simulink model "VendingMachine"  (R2018a)
settings: Solver=FixedStepDiscrete  StartTime=0.0  StopTime=1000  FixedStep=0.1  RelTol=1e-3  EnableMultiTasking=on
settings Model: Creator=higashit  LastModifiedBy=tliang
settings SolverCC: AlgebraicLoopSolver=LineSearch
settings DataIOCC: LimitDataPoints=on  SaveFormat=Array
settings OptimizationCC: DefaultParameterBehavior=Inlined  InlineInvariantSignals=on  ExpressionDepthLimit=2147483647  EfficientFloat2IntCast=on  LifeSpan=inf
settings DebuggingCC: SolverPrmCheckMsg=warning  UniqueDataStoreMsg=error  StateNameClashWarn=warning  StrictBusMsg=ErrorOnBusTreatedAsVector  SFUnexpectedBacktrackingDiag=warning  SFNoUnconditionalDefaultTransitionDiag=warning  SFExecutionAtInitializationDiag=none
settings HardwareCC: ProdBitPerPointer=32  ProdBitPerSizeT=32  ProdBitPerPtrDiffT=32  ProdLargestAtomicFloat=None  ProdIntDivRoundTo=Undefined  ProdEndianess=Unspecified  ProdWordSize=32  ProdHWDeviceType=32-bit Generic
settings ModelReferenceCC: PropagateSignalLabelsOutOfModel=off
settings CodeAppCC: StateflowObjectComments=on
settings GRTTargetCC: TargetLangStandard=C89/C90 (ANSI)  GeneratePreprocessorConditionals=Disable all
settings ConfigComp: CovMetricSettings=dw  CovHtmlReporting=on  CovSaveCumulativeToWorkspaceVar=on  CovSaveSingleToWorkspaceVar=on  CovExternalEMLEnable=off

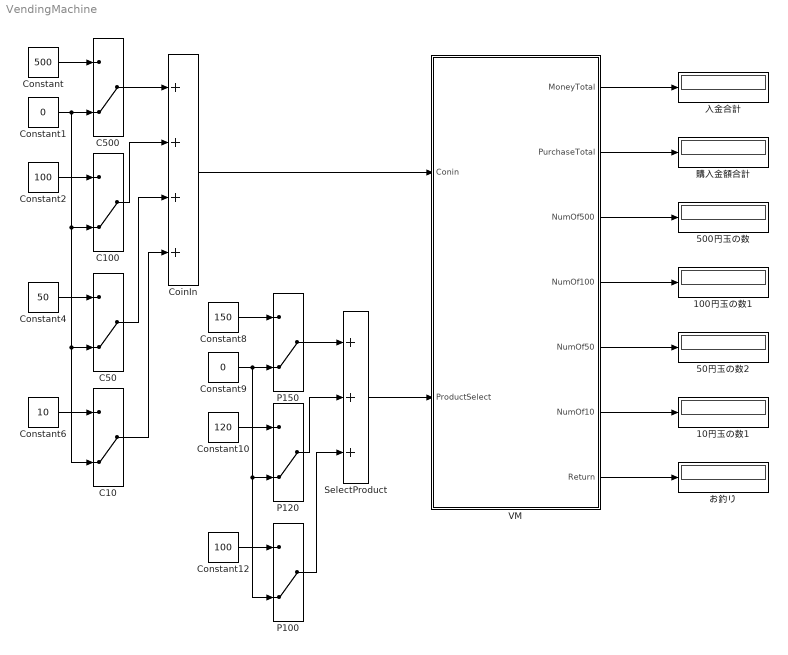
== system VendingMachine ==
  100円玉の数1 : Display
  10円玉の数1 : Display
  500円玉の数 : Display
  50円玉の数2 : Display
  C{10,50,100,500} (4 alike) : ManualSwitch  CurrentSetting=0
  CoinIn : Sum  Inputs=++++
  Constant : Constant  Value=500
  Constant1 : Constant  Value=0
  Constant10 : Constant  Value=120
  Constant12 : Constant  Value=100
  Constant2 : Constant  Value=100
  Constant4 : Constant  Value=50
  Constant6 : Constant  Value=10
  Constant8 : Constant  Value=150
  Constant9 : Constant  Value=0
  P100 : ManualSwitch  CurrentSetting=0
  P120 : ManualSwitch  CurrentSetting=0
  P150 : ManualSwitch  CurrentSetting=0
  SelectProduct : Sum  Inputs=+++
  VM : Subsystem
  お釣り : Display
  入金合計 : Display
  購入金額合計 : Display
  wires:
  Constant8/1 -> P150/1
  Constant9/1 -> P100/2, P120/2, P150/2
  Constant10/1 -> P120/1
  Constant12/1 -> P100/1
  P150/1 -> SelectProduct/1
  P120/1 -> SelectProduct/2
  P100/1 -> SelectProduct/3
  SelectProduct/1 -> VM/2(ProductSelect)
  VM/1(MoneyTotal) -> 入金合計/1
  VM/7(Return) -> お釣り/1
  VM/3(NumOf500) -> 500円玉の数/1
  VM/4(NumOf100) -> 100円玉の数1/1
  VM/5(NumOf50) -> 50円玉の数2/1
  VM/6(NumOf10) -> 10円玉の数1/1
  VM/2(PurchaseTotal) -> 購入金額合計/1
  Constant/1 -> C500/1
  Constant1/1 -> C10/2, C50/2, C100/2, C500/2
  Constant2/1 -> C100/1
  Constant4/1 -> C50/1
  Constant6/1 -> C10/1
  C500/1 -> CoinIn/1
  C100/1 -> CoinIn/2
  C50/1 -> CoinIn/3
  C10/1 -> CoinIn/4
  CoinIn/1 -> VM/1(Conin)

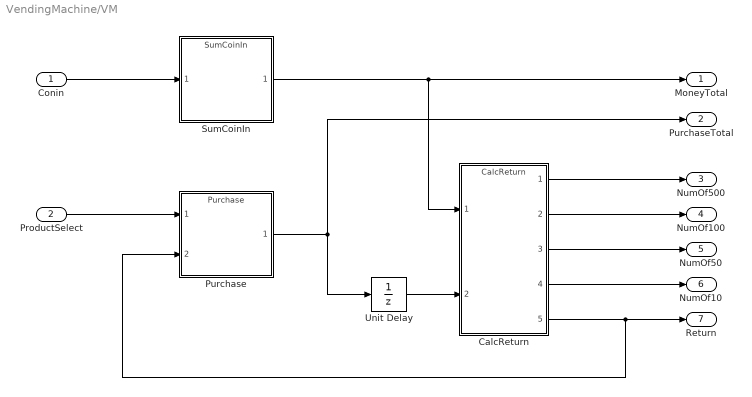
== system VendingMachine/VM ==
  Conin : Inport
  ProductSelect : Inport  Port=2
  CalcReturn : ModelReference  ModelNameDialog=CalcReturn.slx  SimulationMode=Normal  ModelReferenceVersion=1.182
  Purchase : ModelReference  ModelNameDialog=Purchase.slx  SimulationMode=Normal  ModelReferenceVersion=1.182
  SumCoinIn : ModelReference  ModelNameDialog=SumCoinIn.slx  SimulationMode=Normal  ModelReferenceVersion=1.181
  Unit Delay : UnitDelay  SampleTime=-1
  MoneyTotal : Outport
  PurchaseTotal : Outport  Port=2
  NumOf500 : Outport  Port=3
  NumOf100 : Outport  Port=4
  NumOf50 : Outport  Port=5
  NumOf10 : Outport  Port=6
  Return : Outport  Port=7
  wires:
  Conin/1 -> SumCoinIn/1
  ProductSelect/1 -> Purchase/1
  CalcReturn/5 -> Purchase/2, Return/1
  CalcReturn/1 -> NumOf500/1
  CalcReturn/2 -> NumOf100/1
  SumCoinIn/1 -> CalcReturn/1, MoneyTotal/1
  CalcReturn/3 -> NumOf50/1
  CalcReturn/4 -> NumOf10/1
  Purchase/1 -> Unit Delay/1, PurchaseTotal/1
  Unit Delay/1 -> CalcReturn/2
